simulink model "gm_inc_enc_v26"  (R2023a)
settings: Solver=FixedStepDiscrete  StartTime=0.0  StopTime=SimulationsDauer  RelTol=1e-3
undefined symbols (not defined in the file or in its folder): CW_CCW_Switch, d_axis_hit_CompareValue, DiscIntNeverNeededParam, f_ISR, IncPerTurn, inital_zero_speed_timeout, n_max, Offset_Position_elec, Offset_Position_mech, OmegaPerOverSampl, Periode, Phase_Delay_A, Phase_Delay_B, PolePair, QuadratureFactor, reciprocal_iterations, T_fpga, T_mech
libraries: hdlmdlgenlib x16, dspsrcs4 x3, dspswit3 x2, spsEdgeDetectorLib x2, simulink_extras x1
(part 2 of 3)

== system gm_inc_enc_v26/IncEnc_V26/digital_filter1 ==
  A : Inport  OutDataTypeStr=boolean  PortDimensions=1  SampleTime=1e-08
  AND : Logic  Inputs=3  AllPortsSameDT=off  OutDataTypeStr=boolean  SampleTime=1e-08
  AND1 : Logic  Inputs=3  AllPortsSameDT=off  OutDataTypeStr=boolean  SampleTime=1e-08
  NOT : Logic  Operator=NOT  Inputs=1  AllPortsSameDT=off  OutDataTypeStr=boolean  SampleTime=1e-08
  NOT1 : Logic  Operator=NOT  Inputs=1  AllPortsSameDT=off  OutDataTypeStr=boolean  SampleTime=1e-08
  NOT2 : Logic  Operator=NOT  Inputs=1  AllPortsSameDT=off  OutDataTypeStr=boolean  SampleTime=1e-08
  Subsystem1 : Subsystem
  rd_0 : Delay  DelayLength=double(2)  InitialCondition=0  SampleTime=1e-08
  rd_{1..4} (4 alike) : Delay  DelayLength=double(1)  InitialCondition=0  SampleTime=1e-08
  Q : Outport  SampleTime=1e-08
  wires:
  AND/1 -> rd_3/1
  AND1/1 -> Subsystem1/2(R)
  NOT/1 -> AND1/1
  NOT1/1 -> AND1/2
  NOT2/1 -> AND1/3
  Subsystem1/1(Q) -> Q/1
  rd_3/1 -> Subsystem1/1(S)
  A/1 -> rd_0/1
  rd_0/1 -> AND/1, rd_1/1
  rd_1/1 -> AND/2, NOT/1, rd_2/1
  rd_2/1 -> AND/3, NOT1/1, rd_4/1
  rd_4/1 -> NOT2/1

== system gm_inc_enc_v26/IncEnc_V26/digital_filter2 ==
  A : Inport  OutDataTypeStr=boolean  PortDimensions=1  SampleTime=1e-08
  AND : Logic  Inputs=3  AllPortsSameDT=off  OutDataTypeStr=boolean  SampleTime=1e-08
  AND1 : Logic  Inputs=3  AllPortsSameDT=off  OutDataTypeStr=boolean  SampleTime=1e-08
  NOT : Logic  Operator=NOT  Inputs=1  AllPortsSameDT=off  OutDataTypeStr=boolean  SampleTime=1e-08
  NOT1 : Logic  Operator=NOT  Inputs=1  AllPortsSameDT=off  OutDataTypeStr=boolean  SampleTime=1e-08
  NOT2 : Logic  Operator=NOT  Inputs=1  AllPortsSameDT=off  OutDataTypeStr=boolean  SampleTime=1e-08
  Subsystem1 : Subsystem
  rd_0 : Delay  DelayLength=double(2)  InitialCondition=0  SampleTime=1e-08
  rd_{1..4} (4 alike) : Delay  DelayLength=double(1)  InitialCondition=0  SampleTime=1e-08
  Q : Outport  SampleTime=1e-08
  wires:
  AND/1 -> rd_3/1
  AND1/1 -> Subsystem1/2(R)
  NOT/1 -> AND1/1
  NOT1/1 -> AND1/2
  NOT2/1 -> AND1/3
  Subsystem1/1(Q) -> Q/1
  rd_3/1 -> Subsystem1/1(S)
  A/1 -> rd_0/1
  rd_0/1 -> AND/1, rd_1/1
  rd_1/1 -> AND/2, NOT/1, rd_2/1
  rd_2/1 -> AND/3, NOT1/1, rd_4/1
  rd_4/1 -> NOT2/1

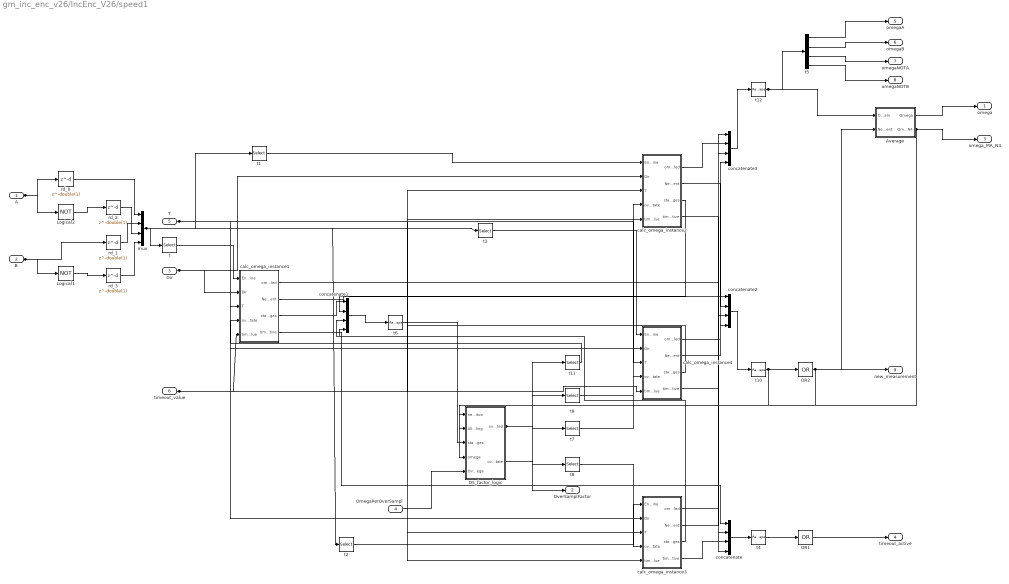
== system gm_inc_enc_v26/IncEnc_V26/speed1 ==
  A : Inport  OutDataTypeStr=boolean  PortDimensions=1  SampleTime=1e-08
  B : Inport  Port=2  OutDataTypeStr=boolean  PortDimensions=1  SampleTime=1e-08
  Dir : Inport  Port=3  OutDataTypeStr=fixdt(1, 4, 0)  PortDimensions=1  SampleTime=1e-08
  OmegaPerOverSampl : Inport  Port=4  OutDataTypeStr=fixdt(1, 24, 11)  PortDimensions=1  SampleTime=1e-08
  T : Inport  Port=5  OutDataTypeStr=fixdt(1, 38, 32)  PortDimensions=1  SampleTime=1e-08
  timeout_value : Inport  Port=6  OutDataTypeStr=uint32  PortDimensions=1  SampleTime=1e-08
  Average : Subsystem
  Logical1 : Logic  Operator=NOT  Inputs=1  AllPortsSameDT=off  OutDataTypeStr=boolean  SampleTime=1e-08
  Logical2 : Logic  Operator=NOT  Inputs=1  AllPortsSameDT=off  OutDataTypeStr=boolean  SampleTime=1e-08
  OR1 : Logic  Operator=OR  Inputs=1  AllPortsSameDT=off  OutDataTypeStr=boolean  SampleTime=1e-08
  OR2 : Logic  Operator=OR  Inputs=1  AllPortsSameDT=off  OutDataTypeStr=boolean  SampleTime=1e-08
  OS_factor_logic : Subsystem
  calc_omega_instance1 : Subsystem
  calc_omega_instance2 : Subsystem
  calc_omega_instance3 : Subsystem
  calc_omega_instance4 : Subsystem
  concatenate{,1..3} (4 alike) : Concatenate  NumInputs=4
  mux : Mux
  rd_{0..3} (4 alike) : Delay  DelayLength=double(1)  InitialCondition=0  SampleTime=1e-08
  t : Selector  SampleTime=1e-08  IndexOptions=Index vector (dialog)  Indices=double(1)  OutputSizes=1
  t1 : Selector  SampleTime=1e-08  IndexOptions=Index vector (dialog)  Indices=double(2)  OutputSizes=1
  t{4,6,10,12} (4 alike) : Reshape
  t11 : Selector  SampleTime=1e-08  IndexOptions=Index vector (dialog)  Indices=double(1)  OutputSizes=1
  t2 : Selector  SampleTime=1e-08  IndexOptions=Index vector (dialog)  Indices=double(3)  OutputSizes=1
  t3 : Selector  SampleTime=1e-08  IndexOptions=Index vector (dialog)  Indices=double(4)  OutputSizes=1
  t5 : Demux
  t7 : Selector  SampleTime=1e-08  IndexOptions=Index vector (dialog)  Indices=double(4)  OutputSizes=1
  t8 : Selector  SampleTime=1e-08  IndexOptions=Index vector (dialog)  Indices=double(3)  OutputSizes=1
  t9 : Selector  SampleTime=1e-08  IndexOptions=Index vector (dialog)  Indices=double(2)  OutputSizes=1
  omega : Outport  SampleTime=1e-08  VectorParamsAs1DForOutWhenUnconnected=off
  OverSamplFactor : Outport  Port=2  SampleTime=1e-08
  omega_MA_N4 : Outport  Port=3  SampleTime=1e-08  VectorParamsAs1DForOutWhenUnconnected=off
  timeout_active : Outport  Port=4  OutDataTypeStr=boolean  SampleTime=1e-08  VectorParamsAs1DForOutWhenUnconnected=off
  omegaA : Outport  Port=5  SampleTime=1e-08  VectorParamsAs1DForOutWhenUnconnected=off
  omegaB : Outport  Port=6  SampleTime=1e-08  VectorParamsAs1DForOutWhenUnconnected=off
  omegaNOTA : Outport  Port=7  SampleTime=1e-08  VectorParamsAs1DForOutWhenUnconnected=off
  omegaNOTB : Outport  Port=8  SampleTime=1e-08  VectorParamsAs1DForOutWhenUnconnected=off
  new_measurement : Outport  Port=9  OutDataTypeStr=boolean  SampleTime=1e-08  VectorParamsAs1DForOutWhenUnconnected=off
  wires:
  A/1 -> rd_0/1, Logical2/1
  B/1 -> rd_1/1, Logical1/1
  Dir/1 -> calc_omega_instance1/2(Dir), calc_omega_instance2/2(Dir), calc_omega_instance3/2(Dir), calc_omega_instance4/2(Dir)
  OmegaPerOverSampl/1 -> OS_factor_logic/5(OverSamplOmega)
  T/1 -> calc_omega_instance1/3(T), calc_omega_instance2/3(T), calc_omega_instance3/3(T), calc_omega_instance4/3(T)
  timeout_value/1 -> calc_omega_instance1/5(timeout_value), calc_omega_instance2/5(timeout_value), calc_omega_instance3/5(timeout_value), calc_omega_instance4/5(timeout_value)
  Average/1(Omega) -> omega/1
  Average/2(OmegaOut_MA_N4) -> omega_MA_N4/1, OS_factor_logic/4(omega)
  Logical1/1 -> rd_3/1
  Logical2/1 -> rd_2/1
  mux/1 -> t3/1, t2/1, t1/1, t/1
  OR1/1 -> timeout_active/1
  OR2/1 -> new_measurement/1, Average/2(NewMeasurement), OS_factor_logic/2(Allow_ToCheckOversampling)
  OS_factor_logic/2(oversampling_state) -> OverSamplFactor/1
  t12/1 -> t5/1, Average/1("OmegaIn ")
  t4/1 -> OR1/1
  t/1 -> calc_omega_instance1/1(Encoder Line)
  t1/1 -> calc_omega_instance2/1(Encoder Line)
  t2/1 -> calc_omega_instance3/1(Encoder Line)
  t3/1 -> calc_omega_instance4/1(Encoder Line)
  concatenate/1 -> t4/1
  calc_omega_instance1/4(timeout_active) -> concatenate/1
  calc_omega_instance2/4(timeout_active) -> concatenate/2
  calc_omega_instance3/4(timeout_active) -> concatenate/3
  calc_omega_instance4/4(timeout_active) -> concatenate/4
  t5/1 -> omegaA/1
  t5/2 -> omegaB/1
  t5/3 -> omegaNOTA/1
  t5/4 -> omegaNOTB/1
  concatenate1/1 -> t6/1
  t6/1 -> OS_factor_logic/3(state_edges)
  t7/1 -> calc_omega_instance4/4(oversampling_state)
  calc_omega_instance4/1(omega_oversampled) -> concatenate3/4
  calc_omega_instance4/2(NewMeasurement) -> concatenate2/4
  calc_omega_instance4/3(state_count_edges) -> concatenate1/4
  t8/1 -> calc_omega_instance3/4(oversampling_state)
  calc_omega_instance3/1(omega_oversampled) -> concatenate3/3
  calc_omega_instance3/2(NewMeasurement) -> concatenate2/3
  calc_omega_instance3/3(state_count_edges) -> concatenate1/3
  t9/1 -> calc_omega_instance2/4(oversampling_state)
  calc_omega_instance2/1(omega_oversampled) -> concatenate3/2
  calc_omega_instance2/2(NewMeasurement) -> concatenate2/2
  calc_omega_instance2/3(state_count_edges) -> concatenate1/2
  concatenate2/1 -> t10/1
  t10/1 -> OR2/1, OS_factor_logic/1(new_transisiton)
  OS_factor_logic/1(oversampling_adjusted) -> t7/1, t8/1, t9/1, t11/1
  t11/1 -> calc_omega_instance1/4(oversampling_state)
  calc_omega_instance1/1(omega_oversampled) -> concatenate3/1
  calc_omega_instance1/2(NewMeasurement) -> concatenate2/1
  calc_omega_instance1/3(state_count_edges) -> concatenate1/1
  concatenate3/1 -> t12/1
  rd_1/1 -> mux/2
  rd_3/1 -> mux/4
  rd_0/1 -> mux/1
  rd_2/1 -> mux/3

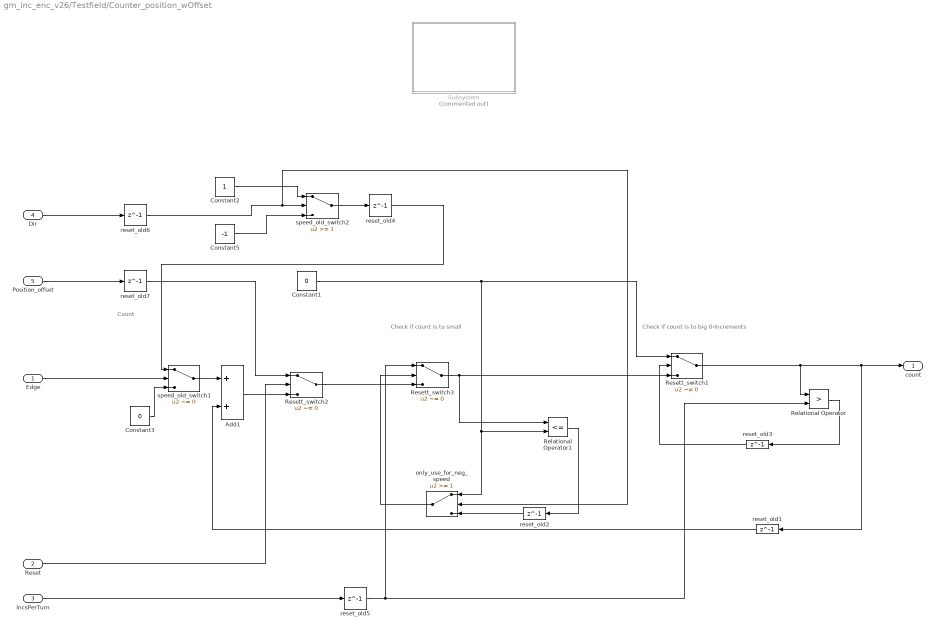
== system gm_inc_enc_v26/Testfield/Counter_position_wOffset ==
  note: Check if count is to big 0-Increments
  note: Count
  note: Check if count is to small
  Edge : Inport
  Reset : Inport  Port=2
  IncsPerTurn : Inport  Port=3
  Dir : Inport  Port=4
  Position_offset : Inport  Port=5
  Add1 : Sum  AccumDataTypeStr=int16  OutDataTypeStr=int16
  Constant1 : Constant  Value=0  OutDataTypeStr=int16  SampleTime=-1
  Constant2 : Constant  OutDataTypeStr=int16  SampleTime=-1
  Constant3 : Constant  Value=0  OutDataTypeStr=int16  SampleTime=-1
  Constant5 : Constant  Value=-1  OutDataTypeStr=int16  SampleTime=-1
  Relational Operator : RelationalOperator  Operator=>  OutDataTypeStr=boolean  InputSameDT=off
  Relational Operator1 : RelationalOperator  Operator=<=  OutDataTypeStr=boolean  InputSameDT=off
  Resett_switch1 : Switch  Criteria=u2 ~= 0  OutDataTypeStr=uint16  SaturateOnIntegerOverflow=off  InputSameDT=off
  Resett_switch2 : Switch  Criteria=u2 ~= 0  OutDataTypeStr=int16  SaturateOnIntegerOverflow=off  InputSameDT=off
  Resett_switch3 : Switch  Criteria=u2 ~= 0  OutDataTypeStr=int16  SaturateOnIntegerOverflow=off  InputSameDT=off
  Subsystem : Subsystem  Commented=on
  only_use_for_neg_speed : Switch  Threshold=1  SaturateOnIntegerOverflow=off  InputSameDT=off
  reset_old{1..7} (7 alike) : Delay  DelayLength=1
  speed_old_switch1 : Switch  Criteria=u2 ~= 0  SaturateOnIntegerOverflow=off  InputSameDT=off
  speed_old_switch2 : Switch  Threshold=1  SaturateOnIntegerOverflow=off  InputSameDT=off
  count : Outport  VectorParamsAs1DForOutWhenUnconnected=off
  wires:
  reset_old7/1 -> Resett_switch2/1
  reset_old6/1 -> speed_old_switch2/2, only_use_for_neg_speed/2
  Dir/1 -> reset_old6/1
  Add1/1 -> Resett_switch2/3
  Position_offset/1 -> reset_old7/1
  reset_old1/1 -> Add1/2
  Edge/1 -> speed_old_switch1/2
  reset_old2/1 -> only_use_for_neg_speed/3
  Reset/1 -> Resett_switch2/2
  IncsPerTurn/1 -> reset_old5/1
  Constant3/1 -> speed_old_switch1/3
  Constant1/1 -> Resett_switch1/1, Relational Operator1/2, only_use_for_neg_speed/1
  Resett_switch1/1 -> reset_old1/1, count/1, Relational Operator/1
  reset_old3/1 -> Resett_switch1/2
  Relational Operator1/1 -> reset_old2/1
  speed_old_switch2/1 -> reset_old4/1
  Resett_switch3/1 -> Resett_switch1/3, Relational Operator1/1
  only_use_for_neg_speed/1 -> Resett_switch3/2
  Resett_switch2/1 -> Resett_switch3/3
  reset_old5/1 -> Relational Operator/2, Resett_switch3/1
  reset_old4/1 -> speed_old_switch1/1
  Constant2/1 -> speed_old_switch2/1
  Relational Operator/1 -> reset_old3/1
  Constant5/1 -> speed_old_switch2/3
  speed_old_switch1/1 -> Add1/1

== system gm_inc_enc_v26/Testfield/Index_Latch ==
  Reset_in : Inport
  Constant : Constant  OutDataTypeStr=boolean
  Constant4 : Constant  Value=0  OutDataTypeStr=boolean
  Delay : Delay  DelayLength=1
  OR : Logic  Operator=OR  AllPortsSameDT=off  OutDataTypeStr=boolean
  Switch : Switch  Criteria=u2 > Threshold  SaturateOnIntegerOverflow=off  InputSameDT=off
  Index_found : Outport
  wires:
  OR/1 -> Switch/2
  Reset_in/1 -> OR/1
  Switch/1 -> Delay/1, Index_found/1
  Constant/1 -> Switch/1
  Delay/1 -> OR/2
  Constant4/1 -> Switch/3

== system gm_inc_enc_v26/Create_Referenz/IncrementalEncoder_Floating/CutTheta_0_2PI ==
  In1 : Inport
  Add7 : Sum  Inputs=+-  OutDataTypeStr=double
  Gain : Gain  Gain=1/(2*pi)
  Gain11 : Gain  Gain=2*pi
  Rounding Function : Rounding
  Out1 : Outport  VectorParamsAs1DForOutWhenUnconnected=off
  wires:
  Add7/1 -> Out1/1
  In1/1 -> Add7/1, Gain/1
  Gain11/1 -> Add7/2
  Rounding Function/1 -> Gain11/1
  Gain/1 -> Rounding Function/1

== system gm_inc_enc_v26/Create_Referenz/IncrementalEncoder_Floating/n_aus_theta_v4 ==
  theta : Inport
  Abs : Abs  SaturateOnIntegerOverflow=off
  Add : Sum  Inputs=-+
  Add1 : Sum  Inputs=+-
  Gain : Gain  Gain=2*pi
  Gain1 : Gain  Gain=1/T_mech
  Gain2 : Gain  Gain=60/(2*pi)
  Geschwindigkeitsfilter1 : Subsystem
  Rate Limiter2 1/T : RateLimiter  RisingSlewLimit=1/T_mech*10  FallingSlewLimit=-1/T_mech*10  SampleTimeMode=inherited
  Saturation : Saturate  UpperLimit=n_max  LowerLimit=-n_max
  Scope1 : Scope  NumInputPorts=5
  Scope2 : Scope  NumInputPorts=5
  Sign : Signum
  Switch : Switch  Threshold=3  SaturateOnIntegerOverflow=off  InputSameDT=off
  Unit Delay : UnitDelay  SampleTime=-1  HasFrameUpgradeWarning=on
  n : Outport  VectorParamsAs1DForOutWhenUnconnected=off
  wires:
  Saturation/1 -> Geschwindigkeitsfilter1/1(In1), Scope1/1
  Rate Limiter2 1/T/1 -> n/1
  Geschwindigkeitsfilter1/1(Out1) -> Rate Limiter2 1/T/1, Scope1/5
  Gain2/1 -> Saturation/1
  Unit Delay/1 -> Add1/2, Scope2/4
  theta/1 -> Unit Delay/1, Add1/1, Scope2/5
  Gain1/1 -> Gain2/1, Scope1/2
  Abs/1 -> Switch/2, Scope1/4
  Add1/1 -> Sign/1, Switch/3, Scope2/2, Abs/1, Add/2, Scope2/3
  Sign/1 -> Gain/1
  Gain/1 -> Add/1
  Add/1 -> Switch/1, Scope2/1
  Switch/1 -> Gain1/1, Scope1/3

== system gm_inc_enc_v26/IncEnc_V26/digital_filter/Subsystem1 ==
  S : Inport  OutDataTypeStr=boolean  PortDimensions=1  SampleTime=1e-08
  R : Inport  Port=2  OutDataTypeStr=boolean  PortDimensions=1  SampleTime=1e-08
  AND : Logic  Operator=NOR  AllPortsSameDT=off  OutDataTypeStr=boolean  SampleTime=1e-08
  AND1 : Logic  Operator=NOR  AllPortsSameDT=off  OutDataTypeStr=boolean  SampleTime=1e-08
  Delay : Delay  DelayLength=double(1)  InitialCondition=0  SampleTime=1e-08
  Q : Outport  SampleTime=1e-08
  wires:
  S/1 -> AND1/2
  R/1 -> AND/1
  AND/1 -> Q/1, Delay/1
  Delay/1 -> AND1/1
  AND1/1 -> AND/2

== system gm_inc_enc_v26/IncEnc_V26/digital_filter1/Subsystem1 ==
  S : Inport  OutDataTypeStr=boolean  PortDimensions=1  SampleTime=1e-08
  R : Inport  Port=2  OutDataTypeStr=boolean  PortDimensions=1  SampleTime=1e-08
  AND : Logic  Operator=NOR  AllPortsSameDT=off  OutDataTypeStr=boolean  SampleTime=1e-08
  AND1 : Logic  Operator=NOR  AllPortsSameDT=off  OutDataTypeStr=boolean  SampleTime=1e-08
  Delay : Delay  DelayLength=double(1)  InitialCondition=0  SampleTime=1e-08
  Q : Outport  SampleTime=1e-08
  wires:
  S/1 -> AND1/2
  R/1 -> AND/1
  AND/1 -> Q/1, Delay/1
  Delay/1 -> AND1/1
  AND1/1 -> AND/2

== system gm_inc_enc_v26/IncEnc_V26/digital_filter2/Subsystem1 ==
  S : Inport  OutDataTypeStr=boolean  PortDimensions=1  SampleTime=1e-08
  R : Inport  Port=2  OutDataTypeStr=boolean  PortDimensions=1  SampleTime=1e-08
  AND : Logic  Operator=NOR  AllPortsSameDT=off  OutDataTypeStr=boolean  SampleTime=1e-08
  AND1 : Logic  Operator=NOR  AllPortsSameDT=off  OutDataTypeStr=boolean  SampleTime=1e-08
  Delay : Delay  DelayLength=double(1)  InitialCondition=0  SampleTime=1e-08
  Q : Outport  SampleTime=1e-08
  wires:
  S/1 -> AND1/2
  R/1 -> AND/1
  AND/1 -> Q/1, Delay/1
  Delay/1 -> AND1/1
  AND1/1 -> AND/2

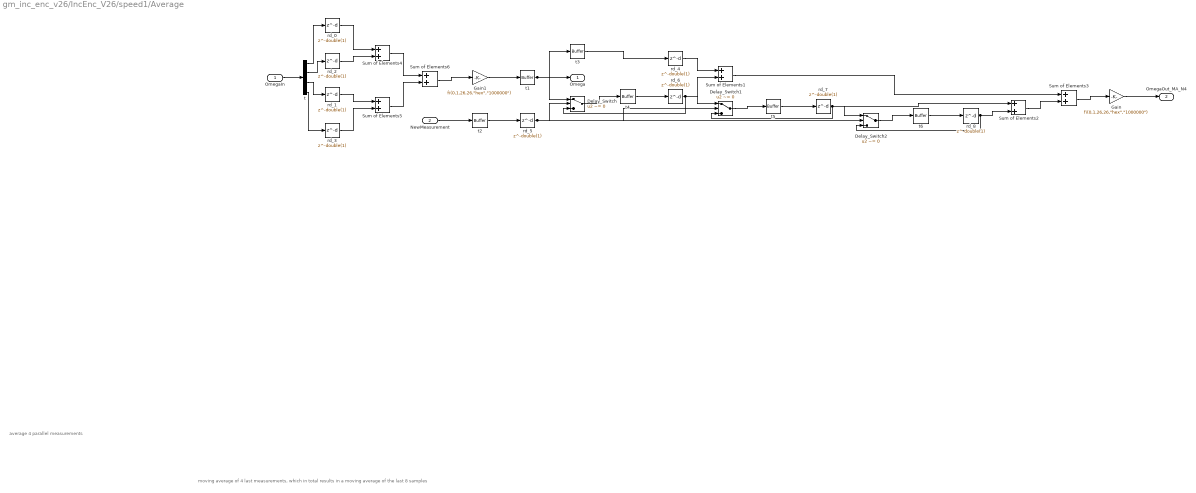
== system gm_inc_enc_v26/IncEnc_V26/speed1/Average ==
  note: moving average of 4 last measurements, which in total results in a moving average of the last 8 samples
  note: average 4 parallel measurements
  "OmegaIn " : Inport  OutDataTypeStr=fixdt(1, 24, 11)  PortDimensions=[4]  SampleTime=1e-08
  NewMeasurement : Inport  Port=2  OutDataTypeStr=boolean  PortDimensions=1  SampleTime=1e-08
  Delay_Switch : Switch  Criteria=u2 ~= 0  Threshold=double(0)  OutDataTypeStr=fixdt(1, 24, 11)  SampleTime=1e-08  SaturateOnIntegerOverflow=off  InputSameDT=off
  Delay_Switch1 : Switch  Criteria=u2 ~= 0  Threshold=double(0)  OutDataTypeStr=fixdt(1, 24, 11)  SampleTime=1e-08  SaturateOnIntegerOverflow=off  InputSameDT=off
  Delay_Switch2 : Switch  Criteria=u2 ~= 0  Threshold=double(0)  OutDataTypeStr=fixdt(1, 24, 11)  SampleTime=1e-08  SaturateOnIntegerOverflow=off  InputSameDT=off
  Gain : Gain  Gain="fi(0,1,26,26,\"hex\",\"1000000\")"  ParamDataTypeStr=fixdt(1, 26, 26)  OutDataTypeStr=fixdt(1, 24, 11)  SampleTime=1e-08
  Gain1 : Gain  Gain="fi(0,1,26,26,\"hex\",\"1000000\")"  ParamDataTypeStr=fixdt(1, 26, 26)  OutDataTypeStr=fixdt(1, 24, 11)  SampleTime=1e-08
  Sum of Elements{1..2,4..5} (4 alike) : Sum  AccumDataTypeStr=fixdt(1, 25, 11)  OutDataTypeStr=fixdt(1, 25, 11)  SampleTime=1e-08
  Sum of Elements3 : Sum  AccumDataTypeStr=fixdt(1, 26, 11)  OutDataTypeStr=fixdt(1, 26, 11)  SampleTime=1e-08
  Sum of Elements6 : Sum  AccumDataTypeStr=fixdt(1, 26, 11)  OutDataTypeStr=fixdt(1, 26, 11)  SampleTime=1e-08
  rd_{0..8} (9 alike) : Delay  DelayLength=double(1)  InitialCondition=0  SampleTime=1e-08
  t : Demux
  t{1..6} (6 alike) : hdlmdlgenlib/Buffer
  Omega : Outport  SampleTime=1e-08  VectorParamsAs1DForOutWhenUnconnected=off
  OmegaOut_MA_N4 : Outport  Port=2  SampleTime=1e-08  VectorParamsAs1DForOutWhenUnconnected=off
  wires:
  t1/1 -> t3/1, Omega/1, Delay_Switch/1
  Gain/1 -> OmegaOut_MA_N4/1
  Gain1/1 -> t1/1
  Sum of Elements1/1 -> Sum of Elements3/1
  Sum of Elements2/1 -> Sum of Elements3/2
  Sum of Elements3/1 -> Gain/1
  Sum of Elements4/1 -> Sum of Elements6/1
  Sum of Elements5/1 -> Sum of Elements6/2
  Sum of Elements6/1 -> Gain1/1
  t3/1 -> rd_4/1
  t/1 -> rd_0/1
  t/2 -> rd_2/1
  t/3 -> rd_1/1
  t/4 -> rd_3/1
  "OmegaIn "/1 -> t/1
  NewMeasurement/1 -> t2/1
  Delay_Switch/1 -> t4/1
  Delay_Switch1/1 -> t5/1
  Delay_Switch2/1 -> t6/1
  rd_0/1 -> Sum of Elements4/1
  rd_2/1 -> Sum of Elements4/2
  rd_3/1 -> Sum of Elements5/2
  rd_1/1 -> Sum of Elements5/1
  rd_4/1 -> Sum of Elements1/1
  t4/1 -> rd_6/1
  rd_6/1 -> Delay_Switch1/1, Delay_Switch/3, Sum of Elements1/2
  t5/1 -> rd_7/1
  rd_7/1 -> Delay_Switch1/3, Delay_Switch2/1, Sum of Elements2/1
  t6/1 -> rd_8/1
  rd_8/1 -> Delay_Switch2/3, Sum of Elements2/2
  t2/1 -> rd_5/1
  rd_5/1 -> Delay_Switch/2, Delay_Switch1/2, Delay_Switch2/2

== system gm_inc_enc_v26/IncEnc_V26/speed1/OS_factor_logic ==
  new_transisiton : Inport  OutDataTypeStr=boolean  PortDimensions=[4]  SampleTime=1e-08
  Allow_ToCheckOversampling : Inport  Port=2  OutDataTypeStr=boolean  PortDimensions=1  SampleTime=1e-08
  state_edges : Inport  Port=3  OutDataTypeStr=int16  PortDimensions=[4]  SampleTime=1e-08
  omega : Inport  Port=4  OutDataTypeStr=fixdt(1, 24, 11)  PortDimensions=1  SampleTime=1e-08
  OverSamplOmega : Inport  Port=5  OutDataTypeStr=fixdt(1, 24, 11)  PortDimensions=1  SampleTime=1e-08
  Abs : Abs  SampleTime=1e-08  OutDataTypeStr=fixdt(1, 24, 11)  SaturateOnIntegerOverflow=off
  Data Type Conversion1 : DataTypeConversion  OutDataTypeStr=fixdt(0,16,0)
  Delay7_Initial_Val : Constant  OutDataTypeStr=uint16  SampleTime=1e-08
  Delay7_ctrl_const : Constant  OutDataTypeStr=boolean  SampleTime=1e-08
  Delay7_switch : Switch  Criteria=u2 ~= 0  Threshold=double(0)  OutDataTypeStr=uint16  SampleTime=1e-08  SaturateOnIntegerOverflow=off  InputSameDT=off
  Sum : Sum  Inputs=+-  AccumDataTypeStr=uint16  OutDataTypeStr=uint16  SampleTime=1e-08
  align_oversamples : Subsystem
  oversample_factor : Subsystem
  rd_{0..3} (4 alike) : Delay  DelayLength=double(1)  InitialCondition=0  SampleTime=1e-08
  oversampling_adjusted : Outport  PortDimensions=4  SampleTime=1e-08
  oversampling_state : Outport  Port=2  SampleTime=1e-08
  wires:
  new_transisiton/1 -> align_oversamples/2(new_transition)
  Allow_ToCheckOversampling/1 -> oversample_factor/1(AllowCheckOverSampl)
  state_edges/1 -> align_oversamples/3(states)
  omega/1 -> Abs/1
  OverSamplOmega/1 -> oversample_factor/3(OverSamplOmega)
  Abs/1 -> oversample_factor/2(ReadBack_Omega)
  Data Type Conversion1/1 -> oversampling_state/1
  Delay7_switch/1 -> Sum/1, Data Type Conversion1/1, oversample_factor/4(state), align_oversamples/1(oversampling_factor)
  Sum/1 -> oversampling_adjusted/1
  align_oversamples/1(delay_output) -> rd_3/1
  oversample_factor/1(state_Out) -> rd_2/1
  oversample_factor/2(InternalOmega_Out) -> rd_1/1
  Delay7_Initial_Val/1 -> Delay7_switch/3
  Delay7_ctrl_const/1 -> rd_0/1
  rd_3/1 -> Sum/2
  rd_2/1 -> Delay7_switch/1
  rd_1/1 -> oversample_factor/5(InternalOmega)
  rd_0/1 -> Delay7_switch/2

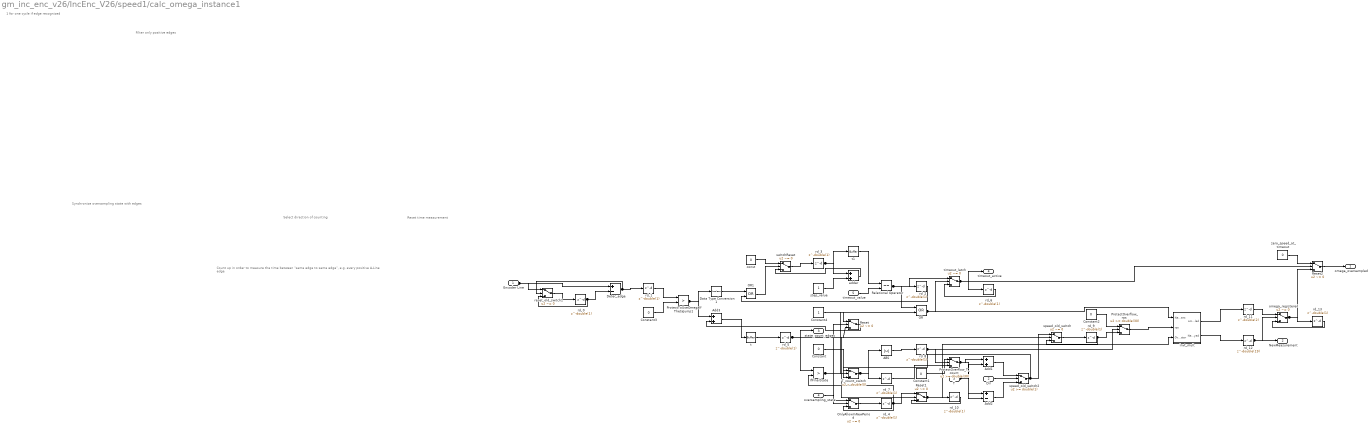
== system gm_inc_enc_v26/IncEnc_V26/speed1/calc_omega_instance1 ==
  note: Count up in order to measure the time between "same edge to same edge", e.g. every positive A-Line edge
  note: Reset time measurement
  note: 1 for one cycle if edge recognized
  note: Select direction of counting
  note: Filter only positive edges
  note: Synchronize oversampling state with edges
  Encoder Line : Inport  OutDataTypeStr=boolean  PortDimensions=1  SampleTime=1e-08
  Dir : Inport  Port=2  OutDataTypeStr=fixdt(1, 4, 0)  PortDimensions=1  SampleTime=1e-08
  T : Inport  Port=3  OutDataTypeStr=fixdt(1, 38, 32)  PortDimensions=1  SampleTime=1e-08
  oversampling_state : Inport  Port=4  OutDataTypeStr=uint16  PortDimensions=1  SampleTime=1e-08
  timeout_value : Inport  Port=5  OutDataTypeStr=uint32  PortDimensions=1  SampleTime=1e-08
  ABS : Abs  SampleTime=1e-08  OutDataTypeStr=fixdt(1, 38, 32)  SaturateOnIntegerOverflow=off
  Add1 : Sum  AccumDataTypeStr=fixdt(1, 38, 32)  OutDataTypeStr=fixdt(1, 38, 32)  SampleTime=1e-08
  Add2 : Sum  Inputs=+-  AccumDataTypeStr=fixdt(1, 38, 32)  OutDataTypeStr=fixdt(1, 38, 32)  SampleTime=1e-08
  Add3 : Sum  AccumDataTypeStr=int16  OutDataTypeStr=int16  SampleTime=1e-08
  Constant : Constant  Value=0  OutDataTypeStr=fixdt(1, 38, 32)  SampleTime=1e-08
  Constant1 : Constant  Value=0  OutDataTypeStr=fixdt(1, 38, 32)  SampleTime=1e-08
  Constant2 : Constant  Value=0  OutDataTypeStr=fixdt(1, 38, 32)  SampleTime=1e-08
  Constant3 : Constant  Value=0  OutDataTypeStr=int8  SampleTime=1e-08
  Constant4 : Constant  OutDataTypeStr=int8  SampleTime=1e-08
  Data Type Conversion1 : DataTypeConversion  OutDataTypeStr=boolean  SampleTime=1e-08  SaturateOnIntegerOverflow=off  RndMeth=Floor
  Detec_edge : Sum  Inputs=+-  AccumDataTypeStr=int8  OutDataTypeStr=int8  SampleTime=1e-08
  IfFinalState : RelationalOperator  Operator=>  OutDataTypeStr=boolean  SampleTime=1e-08  InputSameDT=off
  OR : Logic  Operator=OR  AllPortsSameDT=off  OutDataTypeStr=boolean  SampleTime=1e-08
  OR1 : Logic  Operator=OR  AllPortsSameDT=off  OutDataTypeStr=boolean  SampleTime=1e-08
  OnlyAllowInNewPeriod : Switch  Criteria=u2 ~= 0  Threshold=double(0)  OutDataTypeStr=uint16  SampleTime=1e-08  SaturateOnIntegerOverflow=off  InputSameDT=off
  ProtectOverflow_T_count : Switch  Threshold=double(30)  OutDataTypeStr=fixdt(1, 38, 32)  SampleTime=1e-08  SaturateOnIntegerOverflow=off  InputSameDT=off
  ProtectOverflow_rps : Switch  Threshold=double(30)  OutDataTypeStr=fixdt(1, 38, 32)  SampleTime=1e-08  SaturateOnIntegerOverflow=off  InputSameDT=off
  ProtectToUseOmegaIfThetaJump1 : RelationalOperator  Operator=>  OutDataTypeStr=fixdt(1,16,0)  SampleTime=1e-08  InputSameDT=off
  Relational Operator : RelationalOperator  Operator===  OutDataTypeStr=boolean  SampleTime=1e-08  InputSameDT=off
  Reset : Switch  Criteria=u2 ~= 0  Threshold=double(0)  OutDataTypeStr=fixdt(1, 24, 11)  SampleTime=1e-08  SaturateOnIntegerOverflow=off  InputSameDT=off
  Reset1 : Switch  Criteria=u2 ~= 0  Threshold=double(0)  OutDataTypeStr=uint16  SampleTime=1e-08  SaturateOnIntegerOverflow=off  InputSameDT=off
  Reset2 : Switch  Criteria=u2 ~= 0  Threshold=double(0)  OutDataTypeStr=fixdt(1, 24, 11)  SampleTime=1e-08  SaturateOnIntegerOverflow=off  InputSameDT=off
  T_count_switch : Switch  Criteria=u2 > Threshold  Threshold=double(0)  OutDataTypeStr=fixdt(1, 38, 32)  SampleTime=1e-08  SaturateOnIntegerOverflow=off  InputSameDT=off
  adder : Sum  AccumDataTypeStr=uint32  OutDataTypeStr=uint32  SampleTime=1e-08
  const : Constant  Value=0  VectorParams1D=off  OutDataTypeStr=uint32  SampleTime=1e-08
  invt_mult : Subsystem
  omega_registered : Switch  Criteria=u2 ~= 0  Threshold=double(0)  OutDataTypeStr=fixdt(1, 24, 11)  SampleTime=1e-08  SaturateOnIntegerOverflow=off  InputSameDT=off
  rd_{0..10,13} (12 alike) : Delay  DelayLength=double(1)  InitialCondition=0  SampleTime=1e-08
  rd_11 : Delay  DelayLength=double(2)  InitialCondition=0  SampleTime=1e-08
  rd_12 : Delay  DelayLength=double(19)  InitialCondition=0  SampleTime=1e-08
  reset_old_switch1 : Switch  Criteria=u2 ~= 0  Threshold=double(0)  OutDataTypeStr=boolean  SampleTime=1e-08  SaturateOnIntegerOverflow=off  InputSameDT=off
  speed_old_switch : Switch  Criteria=u2 ~= 0  Threshold=double(0)  OutDataTypeStr=fixdt(1, 38, 32)  SampleTime=1e-08  SaturateOnIntegerOverflow=off  InputSameDT=off
  speed_old_switch2 : Switch  Threshold=double(1)  OutDataTypeStr=fixdt(1, 38, 32)  SampleTime=1e-08  SaturateOnIntegerOverflow=off  InputSameDT=off
  step_value : Constant  VectorParams1D=off  OutDataTypeStr=uint32  SampleTime=1e-08
  switchReset : Switch  Criteria=u2 ~= 0  Threshold=double(0)  OutDataTypeStr=uint32  SampleTime=1e-08  SaturateOnIntegerOverflow=off  InputSameDT=off
  t : hdlmdlgenlib/Buffer
  t1 : hdlmdlgenlib/Buffer
  timeout_latch : Switch  Criteria=u2 ~= 0  Threshold=double(0)  OutDataTypeStr=boolean  SampleTime=1e-08  SaturateOnIntegerOverflow=off  InputSameDT=off
  zero_speed_at_timeout : Constant  Value=0  OutDataTypeStr=fixdt(1, 24, 11)  SampleTime=1e-08
  omega_oversampled : Outport  SampleTime=1e-08  VectorParamsAs1DForOutWhenUnconnected=off
  NewMeasurement : Outport  Port=2  SampleTime=1e-08  VectorParamsAs1DForOutWhenUnconnected=off
  state_count_edges : Outport  Port=3  SampleTime=1e-08  VectorParamsAs1DForOutWhenUnconnected=off
  timeout_active : Outport  Port=4  OutDataTypeStr=boolean  SampleTime=1e-08  VectorParamsAs1DForOutWhenUnconnected=off
  wires:
  rd_4/1 -> Reset1/1, IfFinalState/2, OnlyAllowInNewPeriod/3
  OnlyAllowInNewPeriod/1 -> rd_4/1
  rd_3/1 -> adder/1, t1/1
  switchReset/1 -> rd_3/1
  rd_0/1 -> Detec_edge/2, reset_old_switch1/3
  reset_old_switch1/1 -> rd_0/1
  rd_8/1 -> ProtectOverflow_T_count/2, ProtectOverflow_rps/2
  ABS/1 -> rd_8/1
  rd_5/1 -> IfFinalState/1, state_count_edges/1, Reset/3
  t/1 -> rd_5/1
  rd_12/1 -> omega_registered/2, NewMeasurement/1
  invt_mult/2(New_Measurement_delayed) -> rd_12/1
  rd_9/1 -> ProtectOverflow_rps/3, speed_old_switch/3
  speed_old_switch/1 -> rd_9/1
  rd_11/1 -> omega_registered/1
  rd_1/1 -> ProtectToUseOmegaIfThetaJump1/1
  rd_6/1 -> timeout_latch/3
  rd_13/1 -> omega_registered/3
  rd_7/1 -> ProtectOverflow_T_count/3
  rd_10/1 -> Reset1/3
  rd_2/1 -> OR1/2
  T_count_switch/1 -> ABS/1, rd_7/1
  Add1/1 -> speed_old_switch2/1
  ProtectOverflow_T_count/1 -> Add2/1, Add1/1
  Add2/1 -> speed_old_switch2/3
  Add3/1 -> t/1
  Reset/1 -> Add3/2
  t1/1 -> Relational Operator/1
  OR1/1 -> switchReset/2
  adder/1 -> switchReset/3
  step_value/1 -> adder/2
  const/1 -> switchReset/1
  Constant/1 -> T_count_switch/1
  Constant1/1 -> ProtectOverflow_T_count/1
  Constant2/1 -> ProtectOverflow_rps/1
  Constant3/1 -> ProtectToUseOmegaIfThetaJump1/2
  Constant4/1 -> Reset/1
  Data Type Conversion1/1 -> OR1/1
  Detec_edge/1 -> reset_old_switch1/2, rd_1/1
  IfFinalState/1 -> Reset1/2, speed_old_switch/2, T_count_switch/2, Reset/2, OnlyAllowInNewPeriod/2, OR/2
  OR/1 -> invt_mult/1(New_Measurement), timeout_latch/2
  ProtectOverflow_rps/1 -> invt_mult/2(rps)
  ProtectToUseOmegaIfThetaJump1/1 -> Add3/1, Data Type Conversion1/1
  Relational Operator/1 -> timeout_latch/1, OR/1, rd_2/1
  Reset1/1 -> invt_mult/3(Oversampling Factor), rd_10/1
  Reset2/1 -> omega_oversampled/1
  invt_mult/1(omega_oversampled) -> rd_11/1
  omega_registered/1 -> Reset2/3, rd_13/1
  speed_old_switch2/1 -> speed_old_switch/1, T_count_switch/3
  timeout_latch/1 -> timeout_active/1, Reset2/2, rd_6/1
  zero_speed_at_timeout/1 -> Reset2/1
  timeout_value/1 -> Relational Operator/2
  oversampling_state/1 -> OnlyAllowInNewPeriod/1
  T/1 -> Add2/2, Add1/2
  Dir/1 -> speed_old_switch2/2
  Encoder Line/1 -> reset_old_switch1/1, Detec_edge/1

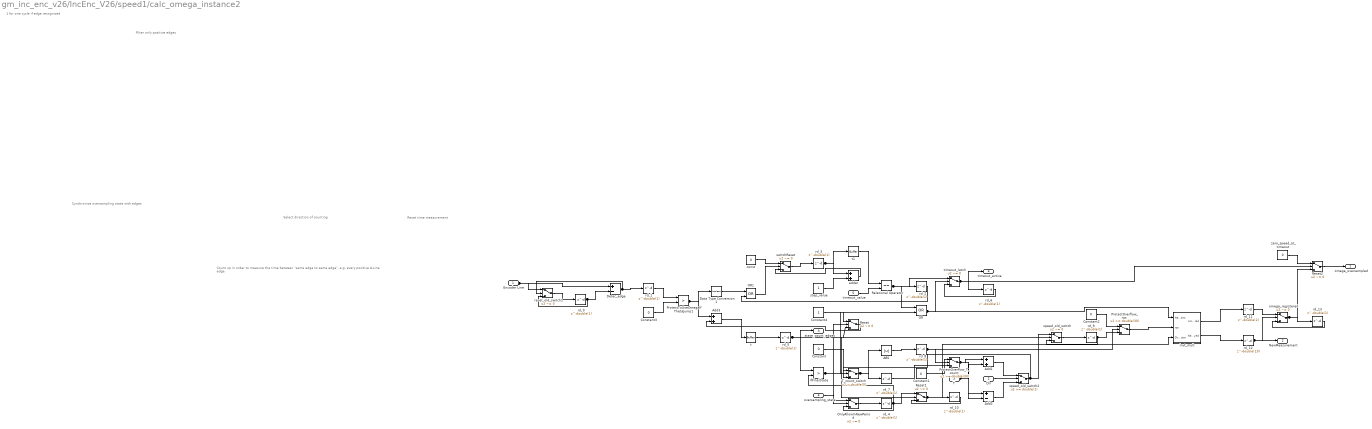
== system gm_inc_enc_v26/IncEnc_V26/speed1/calc_omega_instance2 ==
  note: Count up in order to measure the time between "same edge to same edge", e.g. every positive A-Line edge
  note: Reset time measurement
  note: 1 for one cycle if edge recognized
  note: Select direction of counting
  note: Filter only positive edges
  note: Synchronize oversampling state with edges
  Encoder Line : Inport  OutDataTypeStr=boolean  PortDimensions=1  SampleTime=1e-08
  Dir : Inport  Port=2  OutDataTypeStr=fixdt(1, 4, 0)  PortDimensions=1  SampleTime=1e-08
  T : Inport  Port=3  OutDataTypeStr=fixdt(1, 38, 32)  PortDimensions=1  SampleTime=1e-08
  oversampling_state : Inport  Port=4  OutDataTypeStr=uint16  PortDimensions=1  SampleTime=1e-08
  timeout_value : Inport  Port=5  OutDataTypeStr=uint32  PortDimensions=1  SampleTime=1e-08
  ABS : Abs  SampleTime=1e-08  OutDataTypeStr=fixdt(1, 38, 32)  SaturateOnIntegerOverflow=off
  Add1 : Sum  AccumDataTypeStr=fixdt(1, 38, 32)  OutDataTypeStr=fixdt(1, 38, 32)  SampleTime=1e-08
  Add2 : Sum  Inputs=+-  AccumDataTypeStr=fixdt(1, 38, 32)  OutDataTypeStr=fixdt(1, 38, 32)  SampleTime=1e-08
  Add3 : Sum  AccumDataTypeStr=int16  OutDataTypeStr=int16  SampleTime=1e-08
  Constant : Constant  Value=0  OutDataTypeStr=fixdt(1, 38, 32)  SampleTime=1e-08
  Constant1 : Constant  Value=0  OutDataTypeStr=fixdt(1, 38, 32)  SampleTime=1e-08
  Constant2 : Constant  Value=0  OutDataTypeStr=fixdt(1, 38, 32)  SampleTime=1e-08
  Constant3 : Constant  Value=0  OutDataTypeStr=int8  SampleTime=1e-08
  Constant4 : Constant  OutDataTypeStr=int8  SampleTime=1e-08
  Data Type Conversion1 : DataTypeConversion  OutDataTypeStr=boolean  SampleTime=1e-08  SaturateOnIntegerOverflow=off  RndMeth=Floor
  Detec_edge : Sum  Inputs=+-  AccumDataTypeStr=int8  OutDataTypeStr=int8  SampleTime=1e-08
  IfFinalState : RelationalOperator  Operator=>  OutDataTypeStr=boolean  SampleTime=1e-08  InputSameDT=off
  OR : Logic  Operator=OR  AllPortsSameDT=off  OutDataTypeStr=boolean  SampleTime=1e-08
  OR1 : Logic  Operator=OR  AllPortsSameDT=off  OutDataTypeStr=boolean  SampleTime=1e-08
  OnlyAllowInNewPeriod : Switch  Criteria=u2 ~= 0  Threshold=double(0)  OutDataTypeStr=uint16  SampleTime=1e-08  SaturateOnIntegerOverflow=off  InputSameDT=off
  ProtectOverflow_T_count : Switch  Threshold=double(30)  OutDataTypeStr=fixdt(1, 38, 32)  SampleTime=1e-08  SaturateOnIntegerOverflow=off  InputSameDT=off
  ProtectOverflow_rps : Switch  Threshold=double(30)  OutDataTypeStr=fixdt(1, 38, 32)  SampleTime=1e-08  SaturateOnIntegerOverflow=off  InputSameDT=off
  ProtectToUseOmegaIfThetaJump1 : RelationalOperator  Operator=>  OutDataTypeStr=fixdt(1,16,0)  SampleTime=1e-08  InputSameDT=off
  Relational Operator : RelationalOperator  Operator===  OutDataTypeStr=boolean  SampleTime=1e-08  InputSameDT=off
  Reset : Switch  Criteria=u2 ~= 0  Threshold=double(0)  OutDataTypeStr=fixdt(1, 24, 11)  SampleTime=1e-08  SaturateOnIntegerOverflow=off  InputSameDT=off
  Reset1 : Switch  Criteria=u2 ~= 0  Threshold=double(0)  OutDataTypeStr=uint16  SampleTime=1e-08  SaturateOnIntegerOverflow=off  InputSameDT=off
  Reset2 : Switch  Criteria=u2 ~= 0  Threshold=double(0)  OutDataTypeStr=fixdt(1, 24, 11)  SampleTime=1e-08  SaturateOnIntegerOverflow=off  InputSameDT=off
  T_count_switch : Switch  Criteria=u2 > Threshold  Threshold=double(0)  OutDataTypeStr=fixdt(1, 38, 32)  SampleTime=1e-08  SaturateOnIntegerOverflow=off  InputSameDT=off
  adder : Sum  AccumDataTypeStr=uint32  OutDataTypeStr=uint32  SampleTime=1e-08
  const : Constant  Value=0  VectorParams1D=off  OutDataTypeStr=uint32  SampleTime=1e-08
  invt_mult : Subsystem
  omega_registered : Switch  Criteria=u2 ~= 0  Threshold=double(0)  OutDataTypeStr=fixdt(1, 24, 11)  SampleTime=1e-08  SaturateOnIntegerOverflow=off  InputSameDT=off
  rd_{0..10,13} (12 alike) : Delay  DelayLength=double(1)  InitialCondition=0  SampleTime=1e-08
  rd_11 : Delay  DelayLength=double(2)  InitialCondition=0  SampleTime=1e-08
  rd_12 : Delay  DelayLength=double(19)  InitialCondition=0  SampleTime=1e-08
  reset_old_switch1 : Switch  Criteria=u2 ~= 0  Threshold=double(0)  OutDataTypeStr=boolean  SampleTime=1e-08  SaturateOnIntegerOverflow=off  InputSameDT=off
  speed_old_switch : Switch  Criteria=u2 ~= 0  Threshold=double(0)  OutDataTypeStr=fixdt(1, 38, 32)  SampleTime=1e-08  SaturateOnIntegerOverflow=off  InputSameDT=off
  speed_old_switch2 : Switch  Threshold=double(1)  OutDataTypeStr=fixdt(1, 38, 32)  SampleTime=1e-08  SaturateOnIntegerOverflow=off  InputSameDT=off
  step_value : Constant  VectorParams1D=off  OutDataTypeStr=uint32  SampleTime=1e-08
  switchReset : Switch  Criteria=u2 ~= 0  Threshold=double(0)  OutDataTypeStr=uint32  SampleTime=1e-08  SaturateOnIntegerOverflow=off  InputSameDT=off
  t : hdlmdlgenlib/Buffer
  t1 : hdlmdlgenlib/Buffer
  timeout_latch : Switch  Criteria=u2 ~= 0  Threshold=double(0)  OutDataTypeStr=boolean  SampleTime=1e-08  SaturateOnIntegerOverflow=off  InputSameDT=off
  zero_speed_at_timeout : Constant  Value=0  OutDataTypeStr=fixdt(1, 24, 11)  SampleTime=1e-08
  omega_oversampled : Outport  SampleTime=1e-08  VectorParamsAs1DForOutWhenUnconnected=off
  NewMeasurement : Outport  Port=2  SampleTime=1e-08  VectorParamsAs1DForOutWhenUnconnected=off
  state_count_edges : Outport  Port=3  SampleTime=1e-08  VectorParamsAs1DForOutWhenUnconnected=off
  timeout_active : Outport  Port=4  OutDataTypeStr=boolean  SampleTime=1e-08  VectorParamsAs1DForOutWhenUnconnected=off
  wires:
  rd_4/1 -> Reset1/1, IfFinalState/2, OnlyAllowInNewPeriod/3
  OnlyAllowInNewPeriod/1 -> rd_4/1
  rd_3/1 -> adder/1, t1/1
  switchReset/1 -> rd_3/1
  rd_0/1 -> Detec_edge/2, reset_old_switch1/3
  reset_old_switch1/1 -> rd_0/1
  rd_8/1 -> ProtectOverflow_T_count/2, ProtectOverflow_rps/2
  ABS/1 -> rd_8/1
  rd_5/1 -> IfFinalState/1, state_count_edges/1, Reset/3
  t/1 -> rd_5/1
  rd_12/1 -> omega_registered/2, NewMeasurement/1
  invt_mult/2(New_Measurement_delayed) -> rd_12/1
  rd_9/1 -> ProtectOverflow_rps/3, speed_old_switch/3
  speed_old_switch/1 -> rd_9/1
  rd_11/1 -> omega_registered/1
  rd_1/1 -> ProtectToUseOmegaIfThetaJump1/1
  rd_6/1 -> timeout_latch/3
  rd_13/1 -> omega_registered/3
  rd_7/1 -> ProtectOverflow_T_count/3
  rd_10/1 -> Reset1/3
  rd_2/1 -> OR1/2
  T_count_switch/1 -> ABS/1, rd_7/1
  Add1/1 -> speed_old_switch2/1
  ProtectOverflow_T_count/1 -> Add2/1, Add1/1
  Add2/1 -> speed_old_switch2/3
  Add3/1 -> t/1
  Reset/1 -> Add3/2
  t1/1 -> Relational Operator/1
  OR1/1 -> switchReset/2
  adder/1 -> switchReset/3
  step_value/1 -> adder/2
  const/1 -> switchReset/1
  Constant/1 -> T_count_switch/1
  Constant1/1 -> ProtectOverflow_T_count/1
  Constant2/1 -> ProtectOverflow_rps/1
  Constant3/1 -> ProtectToUseOmegaIfThetaJump1/2
  Constant4/1 -> Reset/1
  Data Type Conversion1/1 -> OR1/1
  Detec_edge/1 -> reset_old_switch1/2, rd_1/1
  IfFinalState/1 -> Reset1/2, speed_old_switch/2, T_count_switch/2, Reset/2, OnlyAllowInNewPeriod/2, OR/2
  OR/1 -> invt_mult/1(New_Measurement), timeout_latch/2
  ProtectOverflow_rps/1 -> invt_mult/2(rps)
  ProtectToUseOmegaIfThetaJump1/1 -> Add3/1, Data Type Conversion1/1
  Relational Operator/1 -> timeout_latch/1, OR/1, rd_2/1
  Reset1/1 -> invt_mult/3(Oversampling Factor), rd_10/1
  Reset2/1 -> omega_oversampled/1
  invt_mult/1(omega_oversampled) -> rd_11/1
  omega_registered/1 -> Reset2/3, rd_13/1
  speed_old_switch2/1 -> speed_old_switch/1, T_count_switch/3
  timeout_latch/1 -> timeout_active/1, Reset2/2, rd_6/1
  zero_speed_at_timeout/1 -> Reset2/1
  timeout_value/1 -> Relational Operator/2
  oversampling_state/1 -> OnlyAllowInNewPeriod/1
  T/1 -> Add2/2, Add1/2
  Dir/1 -> speed_old_switch2/2
  Encoder Line/1 -> reset_old_switch1/1, Detec_edge/1

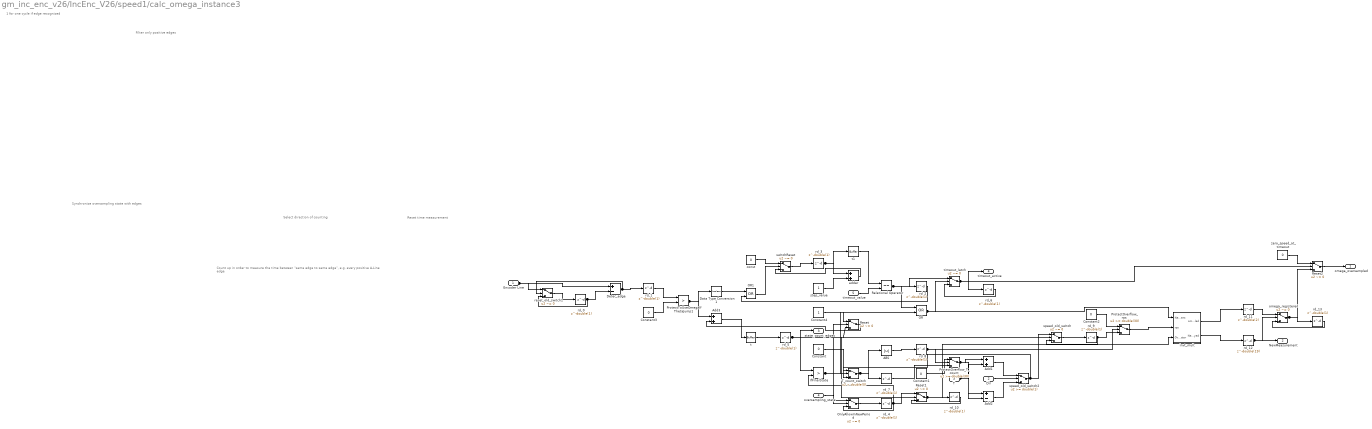
== system gm_inc_enc_v26/IncEnc_V26/speed1/calc_omega_instance3 ==
  note: Count up in order to measure the time between "same edge to same edge", e.g. every positive A-Line edge
  note: Reset time measurement
  note: 1 for one cycle if edge recognized
  note: Select direction of counting
  note: Filter only positive edges
  note: Synchronize oversampling state with edges
  Encoder Line : Inport  OutDataTypeStr=boolean  PortDimensions=1  SampleTime=1e-08
  Dir : Inport  Port=2  OutDataTypeStr=fixdt(1, 4, 0)  PortDimensions=1  SampleTime=1e-08
  T : Inport  Port=3  OutDataTypeStr=fixdt(1, 38, 32)  PortDimensions=1  SampleTime=1e-08
  oversampling_state : Inport  Port=4  OutDataTypeStr=uint16  PortDimensions=1  SampleTime=1e-08
  timeout_value : Inport  Port=5  OutDataTypeStr=uint32  PortDimensions=1  SampleTime=1e-08
  ABS : Abs  SampleTime=1e-08  OutDataTypeStr=fixdt(1, 38, 32)  SaturateOnIntegerOverflow=off
  Add1 : Sum  AccumDataTypeStr=fixdt(1, 38, 32)  OutDataTypeStr=fixdt(1, 38, 32)  SampleTime=1e-08
  Add2 : Sum  Inputs=+-  AccumDataTypeStr=fixdt(1, 38, 32)  OutDataTypeStr=fixdt(1, 38, 32)  SampleTime=1e-08
  Add3 : Sum  AccumDataTypeStr=int16  OutDataTypeStr=int16  SampleTime=1e-08
  Constant : Constant  Value=0  OutDataTypeStr=fixdt(1, 38, 32)  SampleTime=1e-08
  Constant1 : Constant  Value=0  OutDataTypeStr=fixdt(1, 38, 32)  SampleTime=1e-08
  Constant2 : Constant  Value=0  OutDataTypeStr=fixdt(1, 38, 32)  SampleTime=1e-08
  Constant3 : Constant  Value=0  OutDataTypeStr=int8  SampleTime=1e-08
  Constant4 : Constant  OutDataTypeStr=int8  SampleTime=1e-08
  Data Type Conversion1 : DataTypeConversion  OutDataTypeStr=boolean  SampleTime=1e-08  SaturateOnIntegerOverflow=off  RndMeth=Floor
  Detec_edge : Sum  Inputs=+-  AccumDataTypeStr=int8  OutDataTypeStr=int8  SampleTime=1e-08
  IfFinalState : RelationalOperator  Operator=>  OutDataTypeStr=boolean  SampleTime=1e-08  InputSameDT=off
  OR : Logic  Operator=OR  AllPortsSameDT=off  OutDataTypeStr=boolean  SampleTime=1e-08
  OR1 : Logic  Operator=OR  AllPortsSameDT=off  OutDataTypeStr=boolean  SampleTime=1e-08
  OnlyAllowInNewPeriod : Switch  Criteria=u2 ~= 0  Threshold=double(0)  OutDataTypeStr=uint16  SampleTime=1e-08  SaturateOnIntegerOverflow=off  InputSameDT=off
  ProtectOverflow_T_count : Switch  Threshold=double(30)  OutDataTypeStr=fixdt(1, 38, 32)  SampleTime=1e-08  SaturateOnIntegerOverflow=off  InputSameDT=off
  ProtectOverflow_rps : Switch  Threshold=double(30)  OutDataTypeStr=fixdt(1, 38, 32)  SampleTime=1e-08  SaturateOnIntegerOverflow=off  InputSameDT=off
  ProtectToUseOmegaIfThetaJump1 : RelationalOperator  Operator=>  OutDataTypeStr=fixdt(1,16,0)  SampleTime=1e-08  InputSameDT=off
  Relational Operator : RelationalOperator  Operator===  OutDataTypeStr=boolean  SampleTime=1e-08  InputSameDT=off
  Reset : Switch  Criteria=u2 ~= 0  Threshold=double(0)  OutDataTypeStr=fixdt(1, 24, 11)  SampleTime=1e-08  SaturateOnIntegerOverflow=off  InputSameDT=off
  Reset1 : Switch  Criteria=u2 ~= 0  Threshold=double(0)  OutDataTypeStr=uint16  SampleTime=1e-08  SaturateOnIntegerOverflow=off  InputSameDT=off
  Reset2 : Switch  Criteria=u2 ~= 0  Threshold=double(0)  OutDataTypeStr=fixdt(1, 24, 11)  SampleTime=1e-08  SaturateOnIntegerOverflow=off  InputSameDT=off
  T_count_switch : Switch  Criteria=u2 > Threshold  Threshold=double(0)  OutDataTypeStr=fixdt(1, 38, 32)  SampleTime=1e-08  SaturateOnIntegerOverflow=off  InputSameDT=off
  adder : Sum  AccumDataTypeStr=uint32  OutDataTypeStr=uint32  SampleTime=1e-08
  const : Constant  Value=0  VectorParams1D=off  OutDataTypeStr=uint32  SampleTime=1e-08
  invt_mult : Subsystem
  omega_registered : Switch  Criteria=u2 ~= 0  Threshold=double(0)  OutDataTypeStr=fixdt(1, 24, 11)  SampleTime=1e-08  SaturateOnIntegerOverflow=off  InputSameDT=off
  rd_{0..10,13} (12 alike) : Delay  DelayLength=double(1)  InitialCondition=0  SampleTime=1e-08
  rd_11 : Delay  DelayLength=double(2)  InitialCondition=0  SampleTime=1e-08
  rd_12 : Delay  DelayLength=double(19)  InitialCondition=0  SampleTime=1e-08
  reset_old_switch1 : Switch  Criteria=u2 ~= 0  Threshold=double(0)  OutDataTypeStr=boolean  SampleTime=1e-08  SaturateOnIntegerOverflow=off  InputSameDT=off
  speed_old_switch : Switch  Criteria=u2 ~= 0  Threshold=double(0)  OutDataTypeStr=fixdt(1, 38, 32)  SampleTime=1e-08  SaturateOnIntegerOverflow=off  InputSameDT=off
  speed_old_switch2 : Switch  Threshold=double(1)  OutDataTypeStr=fixdt(1, 38, 32)  SampleTime=1e-08  SaturateOnIntegerOverflow=off  InputSameDT=off
  step_value : Constant  VectorParams1D=off  OutDataTypeStr=uint32  SampleTime=1e-08
  switchReset : Switch  Criteria=u2 ~= 0  Threshold=double(0)  OutDataTypeStr=uint32  SampleTime=1e-08  SaturateOnIntegerOverflow=off  InputSameDT=off
  t : hdlmdlgenlib/Buffer
  t1 : hdlmdlgenlib/Buffer
  timeout_latch : Switch  Criteria=u2 ~= 0  Threshold=double(0)  OutDataTypeStr=boolean  SampleTime=1e-08  SaturateOnIntegerOverflow=off  InputSameDT=off
  zero_speed_at_timeout : Constant  Value=0  OutDataTypeStr=fixdt(1, 24, 11)  SampleTime=1e-08
  omega_oversampled : Outport  SampleTime=1e-08  VectorParamsAs1DForOutWhenUnconnected=off
  NewMeasurement : Outport  Port=2  SampleTime=1e-08  VectorParamsAs1DForOutWhenUnconnected=off
  state_count_edges : Outport  Port=3  SampleTime=1e-08  VectorParamsAs1DForOutWhenUnconnected=off
  timeout_active : Outport  Port=4  OutDataTypeStr=boolean  SampleTime=1e-08  VectorParamsAs1DForOutWhenUnconnected=off
  wires:
  rd_4/1 -> Reset1/1, IfFinalState/2, OnlyAllowInNewPeriod/3
  OnlyAllowInNewPeriod/1 -> rd_4/1
  rd_3/1 -> adder/1, t1/1
  switchReset/1 -> rd_3/1
  rd_0/1 -> Detec_edge/2, reset_old_switch1/3
  reset_old_switch1/1 -> rd_0/1
  rd_8/1 -> ProtectOverflow_T_count/2, ProtectOverflow_rps/2
  ABS/1 -> rd_8/1
  rd_5/1 -> IfFinalState/1, state_count_edges/1, Reset/3
  t/1 -> rd_5/1
  rd_12/1 -> omega_registered/2, NewMeasurement/1
  invt_mult/2(New_Measurement_delayed) -> rd_12/1
  rd_9/1 -> ProtectOverflow_rps/3, speed_old_switch/3
  speed_old_switch/1 -> rd_9/1
  rd_11/1 -> omega_registered/1
  rd_1/1 -> ProtectToUseOmegaIfThetaJump1/1
  rd_6/1 -> timeout_latch/3
  rd_13/1 -> omega_registered/3
  rd_7/1 -> ProtectOverflow_T_count/3
  rd_10/1 -> Reset1/3
  rd_2/1 -> OR1/2
  T_count_switch/1 -> ABS/1, rd_7/1
  Add1/1 -> speed_old_switch2/1
  ProtectOverflow_T_count/1 -> Add2/1, Add1/1
  Add2/1 -> speed_old_switch2/3
  Add3/1 -> t/1
  Reset/1 -> Add3/2
  t1/1 -> Relational Operator/1
  OR1/1 -> switchReset/2
  adder/1 -> switchReset/3
  step_value/1 -> adder/2
  const/1 -> switchReset/1
  Constant/1 -> T_count_switch/1
  Constant1/1 -> ProtectOverflow_T_count/1
  Constant2/1 -> ProtectOverflow_rps/1
  Constant3/1 -> ProtectToUseOmegaIfThetaJump1/2
  Constant4/1 -> Reset/1
  Data Type Conversion1/1 -> OR1/1
  Detec_edge/1 -> reset_old_switch1/2, rd_1/1
  IfFinalState/1 -> Reset1/2, speed_old_switch/2, T_count_switch/2, Reset/2, OnlyAllowInNewPeriod/2, OR/2
  OR/1 -> invt_mult/1(New_Measurement), timeout_latch/2
  ProtectOverflow_rps/1 -> invt_mult/2(rps)
  ProtectToUseOmegaIfThetaJump1/1 -> Add3/1, Data Type Conversion1/1
  Relational Operator/1 -> timeout_latch/1, OR/1, rd_2/1
  Reset1/1 -> invt_mult/3(Oversampling Factor), rd_10/1
  Reset2/1 -> omega_oversampled/1
  invt_mult/1(omega_oversampled) -> rd_11/1
  omega_registered/1 -> Reset2/3, rd_13/1
  speed_old_switch2/1 -> speed_old_switch/1, T_count_switch/3
  timeout_latch/1 -> timeout_active/1, Reset2/2, rd_6/1
  zero_speed_at_timeout/1 -> Reset2/1
  timeout_value/1 -> Relational Operator/2
  oversampling_state/1 -> OnlyAllowInNewPeriod/1
  T/1 -> Add2/2, Add1/2
  Dir/1 -> speed_old_switch2/2
  Encoder Line/1 -> reset_old_switch1/1, Detec_edge/1
